simulink model "msePardolMuxOfTwo"  (R2024b)
settings: Solver=VariableStepAuto  StartTime=0.0  StopTime=10.0  RelTol=1e-3
settings Model: Creator=DarianMuresan  LastModifiedBy=ferbe
settings RTWCC: GPUComputeCapability=3.5

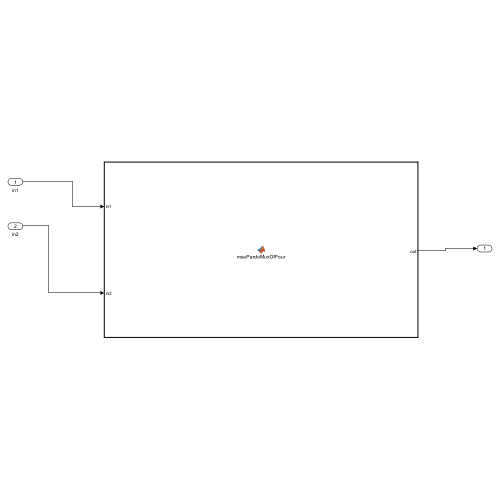
[thumbnail: Simulink's stored preview of the top-level diagram]
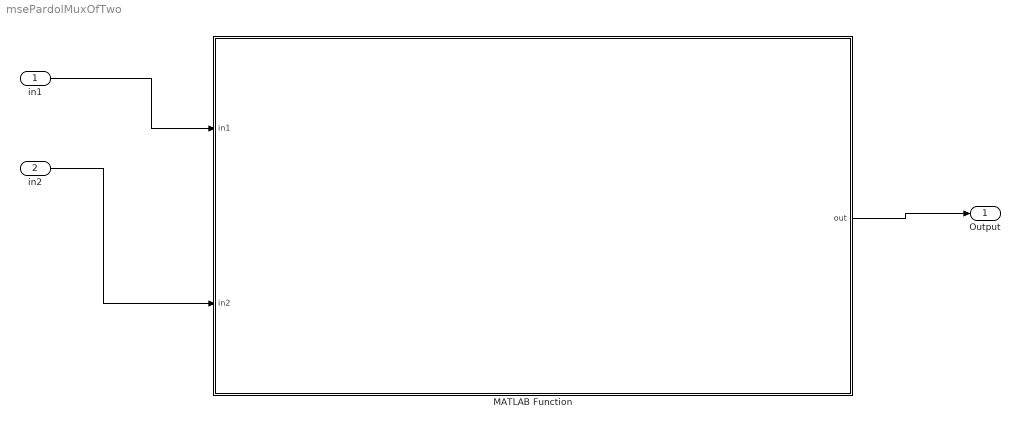
== system msePardolMuxOfTwo ==
  in1 : Inport
  in2 : Inport  Port=2
  MATLAB Function : MATLAB Function  TreatAsAtomicUnit=on
  Output : Outport
  wires:
  in2/1 -> MATLAB Function/2(in2)
  in1/1 -> MATLAB Function/1(in1)
  MATLAB Function/1(out) -> Output/1

== matlab function msePardolMuxOfTwo/MATLAB Function ==
  data: in1 input; out output; in2 input
function out = msePardoMuxOfFour(in1,in2)

% Method to mux 4 inputs from a parallel process.
%
% Written by: Darian Muresan
% Last Modified: 10/10/2024

if nargin<2
    in2=-1;
end

inVector = [in1, in2];

filtered = inVector(inVector > 0);

if isempty(filtered)
    out = -1;
else
    out = max(inVector(inVector>0));
end
